simulink model "CusakisME4901arcs2"  (R2013a)
settings: Solver=ode4  StartTime=0.0  StopTime=inf  FixedStep=0.01  RelTol=1e-3
InitFcn:
  | start_EEVSCube2
  | 
  | %links masses
  | 
  | m=20;%Kg
  | 
  | l=1;%meter
  | 
  | w=0.08;
  | 
  | I=(1/12)*m*(l^2); %moment of inertia
  | 
  | %estimation error
  | 
  | mn=20+m*0.05;
  | In=I+I*0.1;
  | 
  | %controls
  | 
  | a=0.7; %singularity positive gain
  | 
  | %Chaser
  | mb=100;%kg
  | lc=2;%meters
  | lb=lc/2;%meter distance 1joint to CM
  | Ib=(1/12)*mb*(lc^2+lc^2);
  | 
  | %Target
  | 
  | mt=750;%kg target mass
  | lt=1;%meter  side lenght
  | It=(1/6)*(lt^2)*mt;
  | 
  | %Target Initial Conitions
  | 
  | x_t=2;
  | y_t=2;
  | theta_t=0.7853;
  | 
  | Init_t=[x_t;y_t;theta_t;0;0;0];
  | Iinv=pinv(eye(3)*It);
StopFcn:
  | figure(1)
  | subplot(2,1,1)
  | hold on
  | plot(time,kinetic,'g')
  | grid on
  | title('Kinetic Energy vs Time')
  | xlabel('Time')
  | ylabel('Kinetic Energy')
  | hold off
  | 
  | subplot(2,1,2)
  | hold on
  | plot(time,power,'g')
  | grid on
  | title('Power Consumption vs Time')
  | xlabel('Time')
  | ylabel('Power')
  | hold off
  | 
  | chasermapping=[-1,1;-1,-1;1,-1;1,1;-1,1];
  | targetmapping=[1.293,2;2,2.707;2.707,2;2,1.293;1.293,2];
  | 
  | figure(3)
  | hold on
  | plot(EEstate(:,1),EEstate(:,2),'g')
  | plot(targetmapping(:,1),targetmapping(:,2),'r')
  | plot(chasermapping(:,1),chasermapping(:,2),'b')
  | grid on
  | title('End Effector Path')
  | xlabel('X Axis (m)')
  | ylabel('Y Axis (m)')
  | hold off
  | 
  | 
  | figure(4)
  | subplot(2,1,1)
  | hold on
  | plot(time,qqd(:,1),'g')
  | plot(time,qqd(:,2),'r')
  | plot(time,qqd(:,3),'b')
  | grid on
  | title('Theta vs Time')
  | xlabel('Time (sec)')
  | ylabel('Theta (rad)')
  | legend( 'Theta1 ' , ' Theta2 ' , ' Theta3')
  | hold off
  | 
  | subplot(2,1,2)
  | hold on
  | plot(time,qqd(:,4),'g')
  | plot(time,qqd(:,5),'r')
  | plot(time,qqd(:,6),'b')
  | grid on
  | legend( 'Omega1 ' , ' Omega2 ', ' Omega3 ' )
  | title('Omega vs Time')
  | xlabel('Time (sec)')
  | ylabel('Omega (rad/s)')
values from neighbouring files (symbols this model uses):
  D = sqrt((Xf(1)-Xi(1))^2+(Xf(2)-Xi(2))^2)    [Arcpaths.m]
undefined symbols (not defined in the file or in its folder): mesh_A, mesh_B, serial
libraries: instrumentlib x5, simulink x3, vrlib x2, dspinverses x1, aerolibanimutils x1
(part 1 of 4)
settings Model: Creator=Grompone  LastModifiedBy=Admin

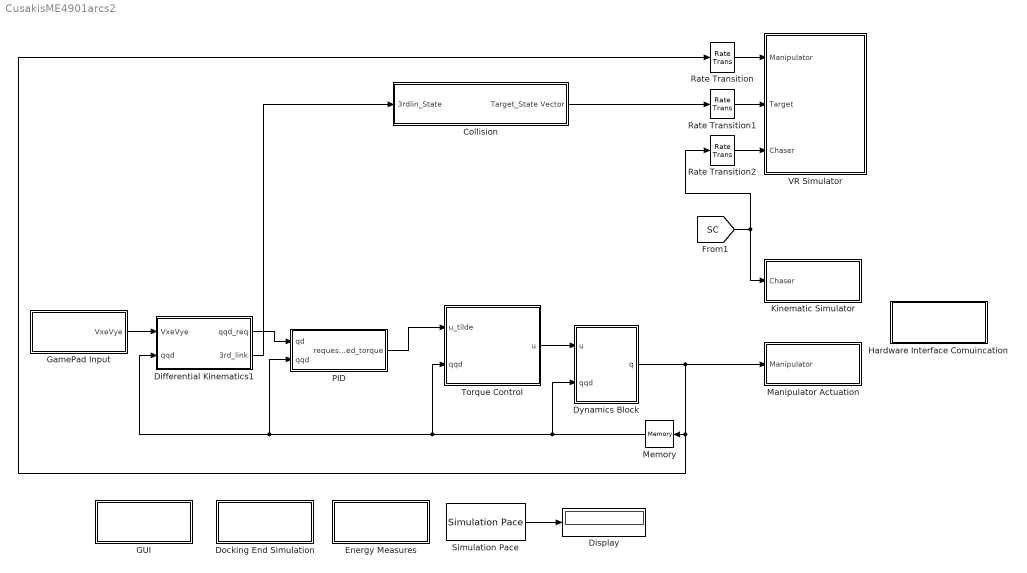
== system CusakisME4901arcs2 ==
  Collision : Subsystem
  Differential Kinematics1 : Subsystem
  Display : Display
  Docking End Simulation : Subsystem
  Dynamics Block : Subsystem
  Energy Measures : Subsystem
  GUI : Subsystem
  GamePad Input : Subsystem
  Hardware Interface Comuincation : Subsystem
  Kinematic Simulator : Subsystem
  Manipulator Actuation : Subsystem
  Memory : Memory  X0=[0 0 0 0 0 0 0 0 0]'
  PID : Subsystem
  Rate Transition : RateTransition  OutPortSampleTime=0.2
  Rate Transition1 : RateTransition  OutPortSampleTime=0.2
  Rate Transition2 : RateTransition  OutPortSampleTime=0.2
  Simulation Pace : aerolibanimutils/Simulation Pace  SimulationPace=1  SleepMode=MATLAB Thread  OutputPaceError=on  SampleTime=0.01
      settings: AttributesFormatString=%<SimulationPace> sec/sec
  Torque Control : Subsystem
  VR Simulator : Subsystem
  wires:
  Torque Control/1(u) -> Dynamics Block/1(u)
  PID/1(requested_torque) -> Torque Control/1(u_tilde)
  Dynamics Block/1(q) -> Manipulator Actuation/1(Manipulator), Rate Transition/1, Memory/1
  Differential Kinematics1/1(qqd_req) -> PID/1(qd)
  GamePad Input/1(VxeVye) -> Differential Kinematics1/1(VxeVye)
  Memory/1 -> Dynamics Block/2(qqd), Torque Control/2(qqd), PID/2(qqd), Differential Kinematics1/2(qqd)
  Collision/1(Target_State Vector) -> Rate Transition1/1
  Differential Kinematics1/2(3rd_link) -> Collision/1(3rdlin_State)
  Rate Transition/1 -> VR Simulator/1(Manipulator)
  Rate Transition1/1 -> VR Simulator/2(Target)
  Rate Transition2/1 -> VR Simulator/3(Chaser)
  Simulation Pace/1 -> Display/1
  [SC] -> Rate Transition2/1, Kinematic Simulator/1(Chaser)

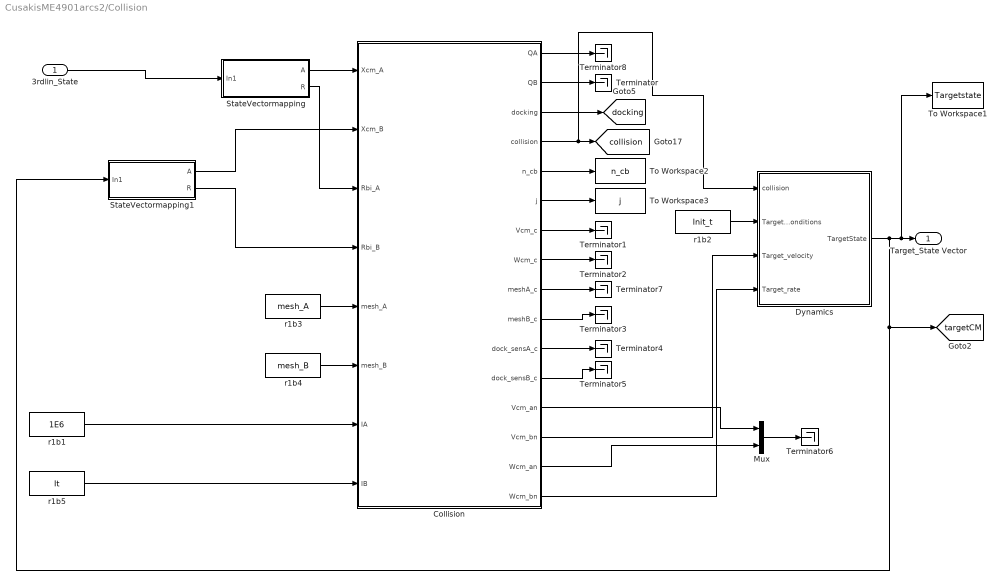
== system CusakisME4901arcs2/Collision ==
  3rdlin_State : Inport
  Collision : Subsystem  mask{mA=1e6, mB=mt, sigma=0.01, sigma_dock=0.25, dotsigma_dock=10, dock_sensA=[0.5 0 0]', dock_sensB=[0 -0.5 0]', epsilon=1}
      mask prompts: mA "Mass of body A [Kg]"; mB "Mass of body B [Kg]"; sigma "Minimum distance for contact [m]"; sigma_dock "Minimum distance for docking (must be greater than contact distance) [m]"; dotsigma_dock "Maximum relative velocity for docking [m/s]"; dock_sensA "Docking sensor position (Body RF) on body A (as [x y z]') [m]"; dock_sensB "Docking sensor position (Body RF) on body B (as [x y z]') [m]"; epsilon "Coefficent of restitution"
      mask help: This block implements collision detection and responce for two rigid bodies of general shapes.
      mask init:
      | ma_mb = [mA; 
      |          mB];
      mask Display:
      | image(imread('collision.jpeg'))
      | color('red');
      | disp('Collision \n Detection and Responce \n v.1.0.9')
      | port_label('input',1,'Xcm_A')
      | port_label('input',2,'Xcm_B')
      | port_label('input',3,'Rbi_A')
      | port_label('input',4,'Rbi_B')
      | port_label('input',5,'mesh_A')
      | port_label('input',6,'mesh_B')
      | port_label('input',7,'IA')
      | port_label('input',8,'IB')
      | 
      | port_label('output',1,'QA')
      | port_label('output',2,'QB')
      | port_label('output',3,'docking')
      | port_label('output',4,'collision')
      | port_label('output',5,'n_cb')
      | port_label('output',6,'j')
      | port_label('output',7,'Vcm_c')
      | port_label('output',8,'Wcm_c')
      | port_label('output',9,'meshA_c')
      | port_label('output',10,'meshB_c')
      | port_label('output',11,'dock_sensA_c')
      | port_label('output',12,'dock_sensB_c')
      | port_label('output',13,'Vcm_an')
      | port_label('output',14,'Vcm_bn')
      | port_label('output',15,'Wcm_an')
      | port_label('output',16,'Wcm_bn')
  Dynamics : Subsystem
  Mux : Mux  Inputs=2
  StateVectormapping : Subsystem
  StateVectormapping1 : Subsystem
  Terminator{,1..8} (9 alike) : Terminator
  To Workspace1 : ToWorkspace  VariableName=Targetstate  SampleTime=-1
  To Workspace2 : ToWorkspace  VariableName=n_cb  SampleTime=-1
  To Workspace3 : ToWorkspace  VariableName=j  SampleTime=-1
  r1b1 : Constant  Value=1E6
  r1b2 : Constant  Value=Init_t
  r1b3 : Constant  Value=mesh_A
  r1b4 : Constant  Value=mesh_B
  r1b5 : Constant  Value=It
  Target_State Vector : Outport
  tag scope: collision=global, docking=global, targetCM=global
  wires:
  Collision/3(docking) -> [docking]
  Collision/6(j) -> To Workspace3/1
  Collision/4(collision) -> Dynamics/1(collision), [collision]
  StateVectormapping/2(R) -> Collision/3(Rbi_A)
  StateVectormapping1/2(R) -> Collision/4(Rbi_B)
  r1b3/1 -> Collision/5(mesh_A)
  r1b4/1 -> Collision/6(mesh_B)
  Collision/5(n_cb) -> To Workspace2/1
  r1b1/1 -> Collision/7(IA)
  Collision/16(Wcm_bn) -> Dynamics/4(Target_rate)
  StateVectormapping1/1(A) -> Collision/2(Xcm_B)
  Collision/14(Vcm_bn) -> Dynamics/3(Target_velocity)
  r1b5/1 -> Collision/8(IB)
  StateVectormapping/1(A) -> Collision/1(Xcm_A)
  Collision/2(QB) -> Terminator/1
  Collision/7(Vcm_c) -> Terminator1/1
  Collision/8(Wcm_c) -> Terminator2/1
  Collision/9(meshA_c) -> Terminator7/1
  Collision/10(meshB_c) -> Terminator3/1
  Collision/11(dock_sensA_c) -> Terminator4/1
  Collision/12(dock_sensB_c) -> Terminator5/1
  Collision/15(Wcm_an) -> Mux/2
  Collision/13(Vcm_an) -> Mux/1
  Collision/1(QA) -> Terminator8/1
  3rdlin_State/1 -> StateVectormapping/1(In1)
  r1b2/1 -> Dynamics/2(Target_InitialConditions)
  Mux/1 -> Terminator6/1
  Dynamics/1(TargetState) -> StateVectormapping1/1(In1), [targetCM], To Workspace1/1, Target_State Vector/1

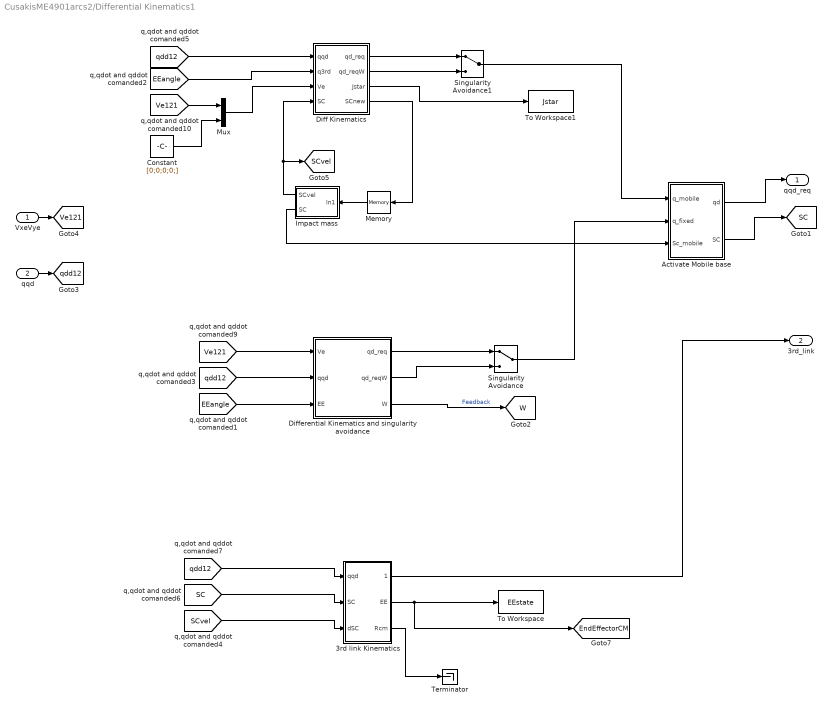
== system CusakisME4901arcs2/Differential Kinematics1 ==
  VxeVye : Inport
  qqd : Inport  Port=2
  3rd link Kinematics : MATLAB Function  TreatAsAtomicUnit=on
  Activate Mobile base : Subsystem
  Constant : Constant  Value=[0;0;0;0;]
  Diff Kinematics : MATLAB Function  TreatAsAtomicUnit=on
  Differential Kinematics and singularity avoidance : MATLAB Function  TreatAsAtomicUnit=on
  Impact mass : Subsystem
  Memory : Memory  X0=[0;0;0;0;0;0]
  Mux : Mux  Inputs=2
  Singularity Avoidance : ManualSwitch
  Singularity Avoidance1 : ManualSwitch
  Terminator : Terminator
  To Workspace : ToWorkspace  VariableName=EEstate  SampleTime=-1
  To Workspace1 : ToWorkspace  VariableName=Jstar  SampleTime=-1
  qqd_req : Outport
  3rd_link : Outport  Port=2
  tag scope: EndEffectorCM=global, SC=global, SCvel=global, Ve121=global, W=global, qdd12=global
  wires:
  Mux/1 -> Diff Kinematics/3(Ve)
  Constant/1 -> Mux/2
  Diff Kinematics/3(Jstar) -> To Workspace1/1
  Memory/1 -> Impact mass/1(In1)
  Diff Kinematics/4(SCnew) -> Memory/1
  Differential Kinematics and singularity avoidance/3(W) -> [W]  "Feedback"
  Differential Kinematics and singularity avoidance/1(qd_req) -> Singularity Avoidance/1
  Differential Kinematics and singularity avoidance/2(qd_reqW) -> Singularity Avoidance/2
  Singularity Avoidance/1 -> Activate Mobile base/2(q_fixed)
  3rd link Kinematics/1(state_3link) -> 3rd_link/1
  3rd link Kinematics/2(EE) -> [EndEffectorCM], To Workspace/1
  qqd/1 -> [qdd12]
  VxeVye/1 -> [Ve121]
  [qdd12] -> Diff Kinematics/1(qqd)
  [SC] -> 3rd link Kinematics/2(SC)
  [qdd12] -> 3rd link Kinematics/1(qqd)
  [qdd12] -> Differential Kinematics and singularity avoidance/2(qqd)
  [Ve121] -> Differential Kinematics and singularity avoidance/1(Ve)
  [EEangle] -> Diff Kinematics/2(q3rd)
  [EEangle] -> Differential Kinematics and singularity avoidance/3(EE)
  [Ve121] -> Mux/1
  Activate Mobile base/1(qd) -> qqd_req/1
  Diff Kinematics/1(qd_req) -> Singularity Avoidance1/1
  Diff Kinematics/2(qd_reqW) -> Singularity Avoidance1/2
  Singularity Avoidance1/1 -> Activate Mobile base/1(q_mobile)
  Impact mass/1(SCvel) -> [SCvel], Diff Kinematics/4(SC)
  Activate Mobile base/2(SC) -> [SC]
  Impact mass/2(SC) -> Activate Mobile base/3(Sc_mobile)
  [SCvel] -> 3rd link Kinematics/3(dSC)
  3rd link Kinematics/3(Rcm) -> Terminator/1

== system CusakisME4901arcs2/Docking End Simulation ==
  Display : Display
  Display1 : Display
  Docking and collision Detection : MATLAB Function  TreatAsAtomicUnit=on
  Memory : Memory
  Stop Simulation : Stop
  tag scope: collcount=global
  wires:
  [docking] -> Docking and collision Detection/1(Docking)
  [collision] -> Docking and collision Detection/3(Collisn)
  [D_Button] -> Docking and collision Detection/2(Dock_button)
  Docking and collision Detection/1(Stop) -> Stop Simulation/1, Display/1
  Docking and collision Detection/2(Count) -> Memory/1, [collcount], Display1/1
  Memory/1 -> Docking and collision Detection/4(Coll)

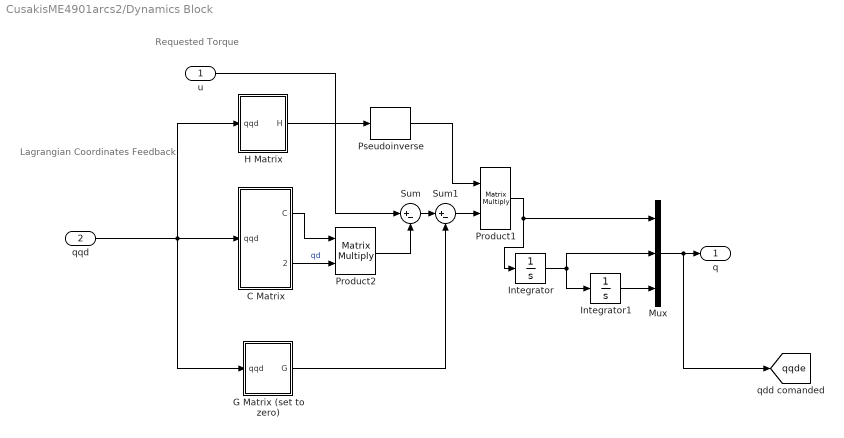
== system CusakisME4901arcs2/Dynamics Block ==
  note: Requested Torque
  note: Lagrangian Coordinates Feedback
  u : Inport
  qqd : Inport  Port=2
  C Matrix : MATLAB Function  TreatAsAtomicUnit=on
  G Matrix (set to zero) : MATLAB Function  TreatAsAtomicUnit=on
  H Matrix : MATLAB Function  TreatAsAtomicUnit=on
  Integrator : Integrator  InitialCondition=[0;0;0]
  Integrator1 : Integrator  InitialCondition=[0;0;0]
  Mux : Mux  Inputs=3
  Product1 : Product  Multiplication=Matrix(*)
  Product2 : Product  Multiplication=Matrix(*)  OutDataTypeStr=int8  LockScale=on
  Pseudoinverse : dspinverses/Pseudoinverse  wanterr=off
  Sum : Sum  Inputs=|+-
  Sum1 : Sum  Inputs=|+-
  q : Outport
  tag scope: qqde=global
  wires:
  Integrator/1 -> Mux/2, Integrator1/1
  Integrator1/1 -> Mux/3
  C Matrix/1(C) -> Product2/1
  H Matrix/1(H) -> Pseudoinverse/1
  Pseudoinverse/1 -> Product1/1
  Product1/1 -> Mux/1, Integrator/1
  Sum/1 -> Sum1/1
  Sum1/1 -> Product1/2
  G Matrix (set to zero)/1(G) -> Sum1/2
  Product2/1 -> Sum/2
  u/1 -> Sum/1
  C Matrix/2(q_dot) -> Product2/2  "qd"
  qqd/1 -> G Matrix (set to zero)/1(qqd), H Matrix/1(qqd), C Matrix/1(qqd)
  Mux/1 -> [qqde], q/1

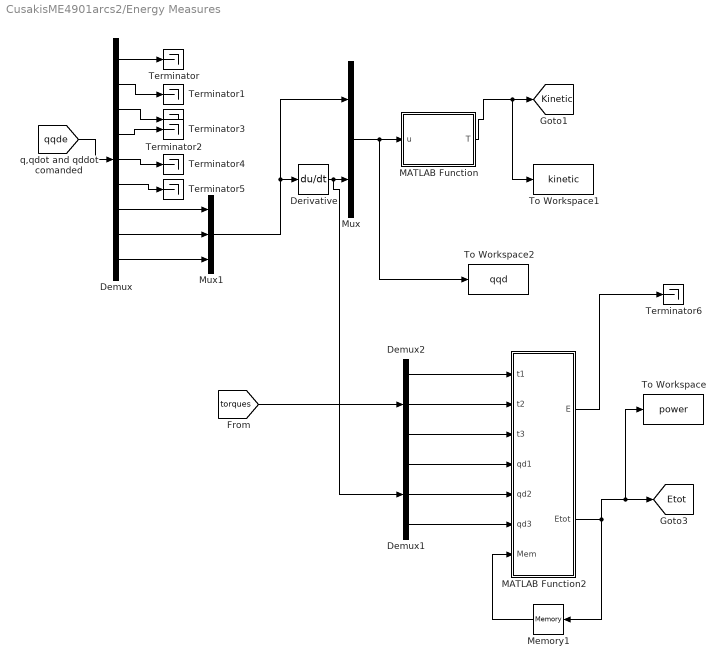
== system CusakisME4901arcs2/Energy Measures ==
  Demux : Demux  Outputs=9
  Demux1 : Demux  Outputs=3
  Demux2 : Demux  Outputs=3
  Derivative : Derivative
  MATLAB Function : MATLAB Function  TreatAsAtomicUnit=on
  MATLAB Function2 : MATLAB Function  TreatAsAtomicUnit=on
  Memory1 : Memory
  Mux : Mux  Inputs=2
  Mux1 : Mux  Inputs=3
  Terminator{,1..6} (7 alike) : Terminator
  To Workspace : ToWorkspace  VariableName=power  SampleTime=-1
  To Workspace1 : ToWorkspace  VariableName=kinetic  SampleTime=-1
  To Workspace2 : ToWorkspace  VariableName=qqd  SampleTime=-1
  tag scope: Etot=global, Kinetic=global
  wires:
  MATLAB Function/1(T) -> To Workspace1/1, [Kinetic]
  [qqde] -> Demux/1
  Demux/1 -> Terminator/1
  Demux/2 -> Terminator1/1
  Demux/3 -> Terminator2/1
  [torques] -> Demux2/1
  Memory1/1 -> MATLAB Function2/7(Mem)
  MATLAB Function2/2(Etot) -> To Workspace/1, [Etot], Memory1/1
  Demux2/1 -> MATLAB Function2/1(t1)
  Demux2/2 -> MATLAB Function2/2(t2)
  Demux2/3 -> MATLAB Function2/3(t3)
  Mux/1 -> To Workspace2/1, MATLAB Function/1(u)
  Demux/7 -> Mux1/1
  Demux/8 -> Mux1/2
  Demux/9 -> Mux1/3
  Demux/4 -> Terminator3/1
  Demux/5 -> Terminator4/1
  Demux/6 -> Terminator5/1
  Mux1/1 -> Derivative/1, Mux/1
  Derivative/1 -> Demux1/1, Mux/2
  Demux1/1 -> MATLAB Function2/4(qd1)
  Demux1/3 -> MATLAB Function2/6(qd3)
  Demux1/2 -> MATLAB Function2/5(qd2)
  MATLAB Function2/1(E) -> Terminator6/1

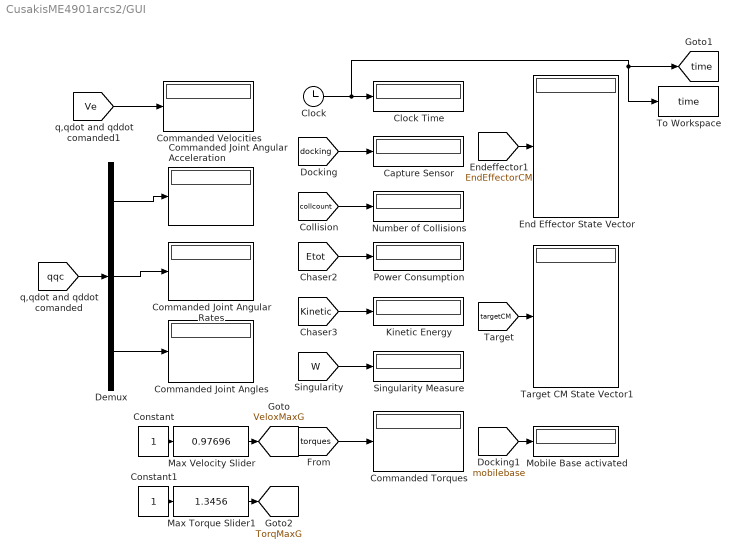
== system CusakisME4901arcs2/GUI ==
  Capture Sensor : Display
  Clock : Clock
  Clock Time : Display
  Commanded Joint Angles : Display
  Commanded Joint Angular Acceleration : Display
  Commanded Joint Angular Rates : Display
  Commanded Torques : Display
  Commanded Velocities : Display
  Constant : Constant
  Constant1 : Constant
  Demux : Demux  Outputs=3
  End Effector State Vector : Display
  Kinetic Energy : Display
  Max Torque Slider1 : simulink/Math Operations/Slider Gain  low=0  gain=1.3456  high=2
  Max Velocity Slider : simulink/Math Operations/Slider Gain  low=0  gain=0.97696  high=2
  Mobile Base activated : Display
  Number of Collisions : Display
  Power Consumption : Display
  Singularity Measure : Display
  Target CM State Vector1 : Display
  To Workspace : ToWorkspace  VariableName=time  SampleTime=-1
  tag scope: TorqMaxG=global, VeloxMaxG=global, time=global
  wires:
  [Ve] -> Commanded Velocities/1
  [W] -> Singularity Measure/1
  [docking] -> Capture Sensor/1
  [collcount] -> Number of Collisions/1
  [qqc] -> Demux/1
  Demux/1 -> Commanded Joint Angular Acceleration/1
  Demux/2 -> Commanded Joint Angular Rates/1
  Demux/3 -> Commanded Joint Angles/1
  [targetCM] -> Target CM State Vector1/1
  [EndEffectorCM] -> End Effector State Vector/1
  [Etot] -> Power Consumption/1
  [Kinetic] -> Kinetic Energy/1
  Constant/1 -> Max Velocity Slider/1
  Max Velocity Slider/1 -> [VeloxMaxG]
  [torques] -> Commanded Torques/1
  Clock/1 -> [time], To Workspace/1, Clock Time/1
  Constant1/1 -> Max Torque Slider1/1
  Max Torque Slider1/1 -> [TorqMaxG]
  [mobilebase] -> Mobile Base activated/1

== system CusakisME4901arcs2/GamePad Input ==
  Joystick Input : vrlib/Joystick Input  joyid=1  adjustports=on  forcefeed=off
  MATLAB Function : MATLAB Function  TreatAsAtomicUnit=on
  Product : Product
  Product1 : Product
  Terminator : Terminator
  VxeVye : Outport
  tag scope: D_Button=global, EEangle=global, Ve=global
  wires:
  Joystick Input/1 -> MATLAB Function/1(Axes)
  Joystick Input/2 -> MATLAB Function/2(Buttons)
  ? -> Terminator/1
  MATLAB Function/2(but) -> [D_Button]
  MATLAB Function/3(j) -> Product1/1
  Product/1 -> VxeVye/1, [Ve]
  [VeloxMaxG] -> Product/2
  MATLAB Function/1(u) -> Product/1
  [TorqMaxG] -> Product1/2
  Product1/1 -> [EEangle]

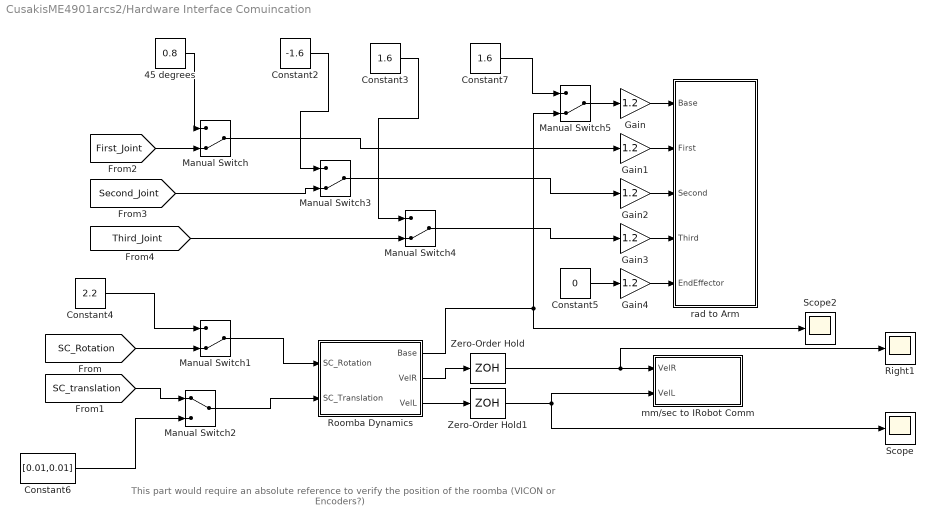
== system CusakisME4901arcs2/Hardware Interface Comuincation ==
  note: This part would require an absolute reference to verify the position of the roomba (VICON or Encoders?)
  45 degrees : Constant  Value=0.8
  Constant2 : Constant  Value=-1.6
  Constant3 : Constant  Value=1.6
  Constant4 : Constant  Value=2.2
  Constant5 : Constant  Value=0
  Constant6 : Constant  Value=[0.01,0.01]
  Constant7 : Constant  Value=1.6
  Gain{,1..4} (5 alike) : Gain  Gain=1.2
  Manual Switch{,1,3..5} (5 alike) : ManualSwitch  CurrentSetting=0
  Manual Switch2 : ManualSwitch
  Right1 : Scope
      settings: SaveName=ScopeData10
  Roomba Dynamics : Subsystem
  Scope : Scope
      settings: SaveName=ScopeData9
  Scope2 : Scope
      settings: SaveName=ScopeData11
  Zero-Order Hold : ZeroOrderHold
  Zero-Order Hold1 : ZeroOrderHold
  mm/sec to IRobot Comm : Subsystem
  rad to Arm : Subsystem
  wires:
  Constant5/1 -> Gain4/1
  [SC_Rotation] -> Manual Switch1/2
  [SC_translation] -> Manual Switch2/1
  Manual Switch2/1 -> Roomba Dynamics/2(SC_Translation)
  [Third_Joint] -> Manual Switch4/2
  Manual Switch4/1 -> Gain3/1
  [Second_Joint] -> Manual Switch3/2
  Manual Switch3/1 -> Gain2/1
  [First_Joint] -> Manual Switch/2
  Manual Switch/1 -> Gain1/1
  45 degrees/1 -> Manual Switch/1
  Constant2/1 -> Manual Switch3/1
  Constant3/1 -> Manual Switch4/1
  Constant4/1 -> Manual Switch1/1
  Constant6/1 -> Manual Switch2/2
  Constant7/1 -> Manual Switch5/1
  Roomba Dynamics/2(VelR) -> Zero-Order Hold/1
  Roomba Dynamics/3(VelL) -> Zero-Order Hold1/1
  Zero-Order Hold/1 -> Right1/1, mm/sec to IRobot Comm/1(VelR)
  Zero-Order Hold1/1 -> mm/sec to IRobot Comm/2(VelL), Scope/1
  Manual Switch5/1 -> Gain/1
  Gain/1 -> rad to Arm/1(Base)
  Gain1/1 -> rad to Arm/2(First)
  Gain2/1 -> rad to Arm/3(Second)
  Gain3/1 -> rad to Arm/4(Third)
  Gain4/1 -> rad to Arm/5(EndEffector)
  Roomba Dynamics/1(Base) -> Scope2/1, Manual Switch5/2
  Manual Switch1/1 -> Roomba Dynamics/1(SC_Rotation)

== system CusakisME4901arcs2/Kinematic Simulator ==
  Chaser : Inport
  Chaser Data : Subsystem
  Scope : Scope
      settings: SaveName=ScopeData3
  Scope2 : Scope
      settings: SaveName=ScopeData4
  chaseCM : Terminator
  tag scope: SC_Rotation=global, SC_translation=global
  wires:
  Chaser/1 -> chaseCM/1, Chaser Data/1(In1)
  Chaser Data/1(Rotation) -> [SC_Rotation], Scope/1
  Chaser Data/2(Translation) -> [SC_translation], Scope2/1

== system CusakisME4901arcs2/Manipulator Actuation ==
  Manipulator : Inport
  Manipulator Joints : Subsystem
  Scope : Scope
  Scope1 : Scope
  Scope2 : Scope
      settings: SaveName=ScopeData2
  tag scope: First_Joint=global, Second_Joint=global, Third_Joint=global
  wires:
  Manipulator/1 -> Manipulator Joints/1(In1)
  Manipulator Joints/1(Joint1) -> Scope/1, [First_Joint]
  Manipulator Joints/3(Joint4) -> [Third_Joint], Scope1/1
  Manipulator Joints/2(Joint3) -> [Second_Joint], Scope2/1

== system CusakisME4901arcs2/PID ==
  qd : Inport
  qqd : Inport  Port=2
  Add : Sum  Inputs=+++
  Demux : Demux  Outputs=3
  Derivative : Derivative
  Gain : Gain
  Gain1 : Gain
  Gain2 : Gain
  Integrator : Integrator  InitialCondition=[0; 0; 0]
  Mux : Mux  Inputs=3
  Sum : Sum  Inputs=|+-
  Sum1 : Sum  Inputs=|+-
  Terminator : Terminator
  requested_torque : Outport
  tag scope: qqc=global
  wires:
  qqd/1 -> Demux/1
  Demux/2 -> Sum/2
  Demux/1 -> Terminator/1
  Sum/1 -> Gain/1
  qd/1 -> Derivative/1, Integrator/1, Sum/1
  Gain/1 -> Mux/2, Add/2
  Sum1/1 -> Gain1/1
  Demux/3 -> Sum1/2
  Add/1 -> requested_torque/1
  Mux/1 -> [qqc]
  Gain1/1 -> Mux/3, Add/3  "Feedback"
  Integrator/1 -> Sum1/1
  Gain2/1 -> Add/1, Mux/1
  Derivative/1 -> Gain2/1

== system CusakisME4901arcs2/Torque Control ==
  u_tilde : Inport
  qqd : Inport  Port=2
  C Matrix : MATLAB Function  TreatAsAtomicUnit=on
  C*q : Product  Multiplication=Matrix(*)
  G Matrix (set zero) : MATLAB Function  TreatAsAtomicUnit=on
  H Matrix : MATLAB Function  TreatAsAtomicUnit=on
  H*u : Product  Multiplication=Matrix(*)
  Subtract : Sum  Inputs=+++
  u : Outport
  tag scope: torques=global
  wires:
  H*u/1 -> Subtract/1
  Subtract/1 -> [torques], u/1
  C*q/1 -> Subtract/2
  C Matrix/1(C) -> C*q/1
  G Matrix (set zero)/1(G) -> Subtract/3
  C Matrix/2(q_dot) -> C*q/2  "qd"
  u_tilde/1 -> H*u/2
  H Matrix/1(H) -> H*u/1
  qqd/1 -> H Matrix/1(qqd), C Matrix/1(qqd), G Matrix (set zero)/1(qqd)

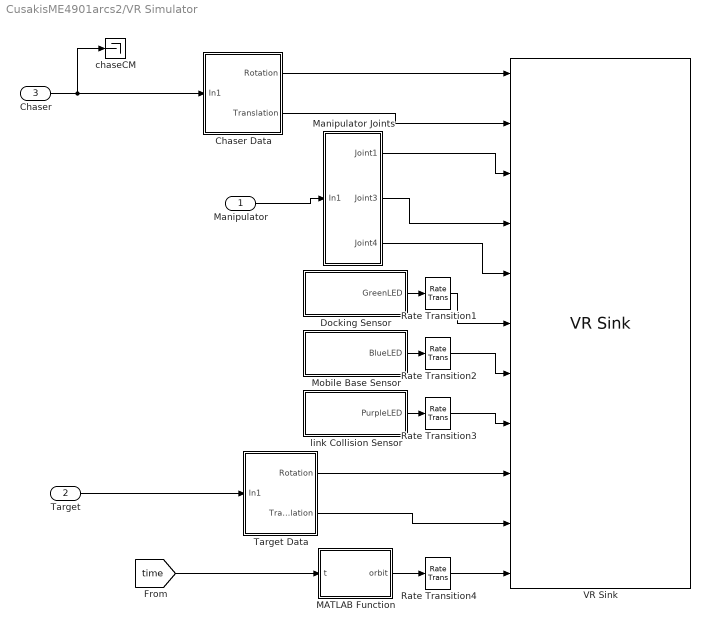
== system CusakisME4901arcs2/VR Simulator ==
  Manipulator : Inport
  Target : Inport  Port=2
  Chaser : Inport  Port=3
  Chaser Data : Subsystem
  Docking Sensor : Subsystem
  MATLAB Function : MATLAB Function  TreatAsAtomicUnit=on
  Manipulator Joints : Subsystem
  Mobile Base Sensor : Subsystem
  Rate Transition{1..4} (4 alike) : RateTransition  OutPortSampleTime=0.2
  Target Data : Subsystem
  VR Sink : vrlib/VR Sink  InstantiateOnLoad=on  SampleTime=0.2  ViewEnable=on  RemoteChange=off  RemoteView=off  FieldsWritten=CHASER.rotation.4.1.1.double#CHASER.translation.3.1.1.double#Joint1.rotation.4.1.1.double#Joint2.rotation.4.1.1.double#Joint3.rotation.4.1.1.double#we.diffuseColor.3.1.1.double#g.diffuseColor.3.1.1.double#Cl.diffuseColor.3.1.1.double#TARGET.rotation.4.1.1.double#TARGET.translation.3.1.1.double#Otherview.translation.3.1.1.double  WorldFileName=final1b.wrl  AutoView=off  VideoDimensions=[]  AllowVariableSize=off
  chaseCM : Terminator
  link Collision Sensor : Subsystem
  wires:
  Manipulator/1 -> Manipulator Joints/1(In1)
  Target/1 -> Target Data/1(In1)
  [time] -> MATLAB Function/1(t)
  Chaser/1 -> chaseCM/1, Chaser Data/1(In1)
  Chaser Data/1(Rotation) -> VR Sink/1
  Chaser Data/2(Translation) -> VR Sink/2
  Manipulator Joints/1(Joint1) -> VR Sink/3
  Manipulator Joints/3(Joint4) -> VR Sink/5
  Target Data/1(Rotation) -> VR Sink/9
  Target Data/2(Translation) -> VR Sink/10
  MATLAB Function/1(orbit) -> Rate Transition4/1
  link Collision Sensor/1(PurpleLED) -> Rate Transition3/1
  Docking Sensor/1(GreenLED) -> Rate Transition1/1
  Mobile Base Sensor/1(BlueLED) -> Rate Transition2/1
  Manipulator Joints/2(Joint3) -> VR Sink/4
  Rate Transition1/1 -> VR Sink/6
  Rate Transition2/1 -> VR Sink/7
  Rate Transition3/1 -> VR Sink/8
  Rate Transition4/1 -> VR Sink/11

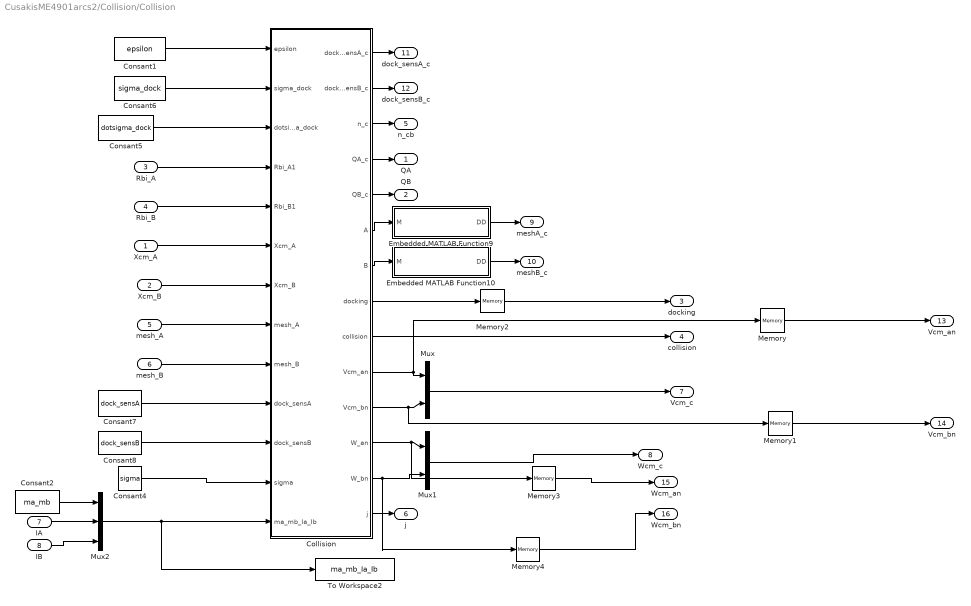
== system CusakisME4901arcs2/Collision/Collision ==
  Xcm_A : Inport
  Xcm_B : Inport  Port=2
  Rbi_A : Inport  Port=3
  Rbi_B : Inport  Port=4
  mesh_A : Inport  Port=5
  mesh_B : Inport  Port=6
  IA : Inport  Port=7
  IB : Inport  Port=8
  Collision : MATLAB Function  TreatAsAtomicUnit=on
  Consant1 : Constant  Value=epsilon
  Consant2 : Constant  Value=ma_mb
  Consant4 : Constant  Value=sigma
  Consant5 : Constant  Value=dotsigma_dock
  Consant6 : Constant  Value=sigma_dock
  Consant7 : Constant  Value=dock_sensA
  Consant8 : Constant  Value=dock_sensB
  Embedded MATLAB Function10 : MATLAB Function  TreatAsAtomicUnit=on
  Embedded MATLAB Function9 : MATLAB Function  TreatAsAtomicUnit=on
  Memory{,1,3..4} (4 alike) : Memory  X0=zeros(3,1)
  Memory2 : Memory
  Mux : Mux  Inputs=2
  Mux1 : Mux  Inputs=2
  Mux2 : Mux  Inputs=3
  To Workspace2 : ToWorkspace  VariableName=ma_mb_Ia_Ib  SampleTime=-1
  QA : Outport
  QB : Outport  Port=2
  docking : Outport  Port=3
  collision : Outport  Port=4
  n_cb : Outport  Port=5
  j : Outport  Port=6
  Vcm_c : Outport  Port=7
  Wcm_c : Outport  Port=8
  meshA_c : Outport  Port=9
  meshB_c : Outport  Port=10
  dock_sensA_c : Outport  Port=11
  dock_sensB_c : Outport  Port=12
  Vcm_an : Outport  Port=13
  Vcm_bn : Outport  Port=14
  Wcm_an : Outport  Port=15
  Wcm_bn : Outport  Port=16
  wires:
  Embedded MATLAB Function9/1(DD) -> meshA_c/1
  Embedded MATLAB Function10/1(DD) -> meshB_c/1
  Collision/6(A) -> Embedded MATLAB Function9/1(M)
  Collision/7(B) -> Embedded MATLAB Function10/1(M)
  Rbi_B/1 -> Collision/5(Rbi_B1)
  Xcm_A/1 -> Collision/6(Xcm_A)
  mesh_A/1 -> Collision/8(mesh_A)
  mesh_B/1 -> Collision/9(mesh_B)
  Collision/3(n_c) -> n_cb/1
  Collision/8(docking) -> Memory2/1
  Collision/10(Vcm_an) -> Mux/1, Memory/1
  Collision/13(W_bn) -> Mux1/2, Memory4/1
  Collision/14(j) -> j/1
  Collision/9(collision) -> collision/1
  Mux/1 -> Vcm_c/1
  Mux1/1 -> Wcm_c/1
  Collision/4(QA_c) -> QA/1
  Collision/5(QB_c) -> QB/1
  Collision/11(Vcm_bn) -> Memory1/1, Mux/2
  Collision/12(W_an) -> Memory3/1, Mux1/1
  Xcm_B/1 -> Collision/7(Xcm_B)
  Collision/2(dock_sensB_c) -> dock_sensB_c/1
  Collision/1(dock_sensA_c) -> dock_sensA_c/1
  Consant4/1 -> Collision/12(sigma)
  Consant5/1 -> Collision/3(dotsigma_dock)
  Rbi_A/1 -> Collision/4(Rbi_A1)
  Consant6/1 -> Collision/2(sigma_dock)
  Consant7/1 -> Collision/10(dock_sensA)
  Consant8/1 -> Collision/11(dock_sensB)
  Consant1/1 -> Collision/1(epsilon)
  Mux2/1 -> Collision/13(ma_mb_Ia_Ib), To Workspace2/1
  Consant2/1 -> Mux2/1
  IA/1 -> Mux2/2
  IB/1 -> Mux2/3
  Memory/1 -> Vcm_an/1
  Memory1/1 -> Vcm_bn/1
  Memory3/1 -> Wcm_an/1
  Memory4/1 -> Wcm_bn/1
  Memory2/1 -> docking/1

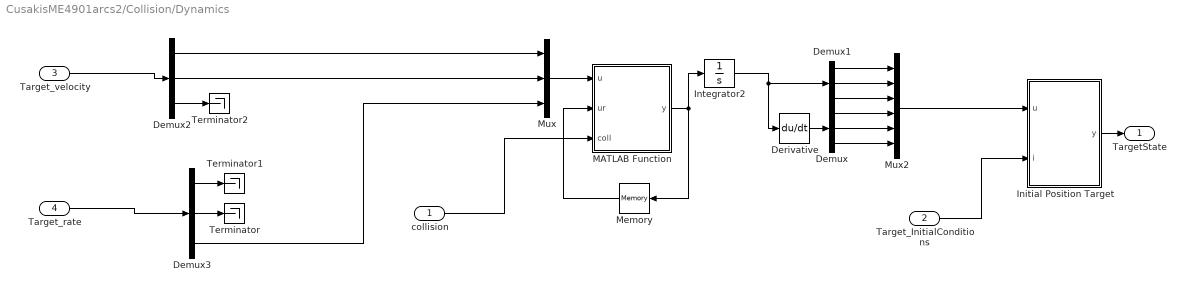
== system CusakisME4901arcs2/Collision/Dynamics ==
  collision : Inport
  Target_InitialConditions : Inport  Port=2
  Target_velocity : Inport  Port=3
  Target_rate : Inport  Port=4
  Demux{,1..3} (4 alike) : Demux  Outputs=3
  Derivative : Derivative
  Initial Position Target : MATLAB Function  TreatAsAtomicUnit=on
  Integrator2 : Integrator
  MATLAB Function : MATLAB Function  TreatAsAtomicUnit=on
  Memory : Memory  X0=[0;0;0]
  Mux : Mux  Inputs=3
  Mux2 : Mux  Inputs=6
  Terminator : Terminator
  Terminator1 : Terminator
  Terminator2 : Terminator
  TargetState : Outport
  wires:
  Target_InitialConditions/1 -> Initial Position Target/2(i)
  Initial Position Target/1(y) -> TargetState/1
  Demux2/1 -> Mux/1
  Demux2/2 -> Mux/2
  Demux3/3 -> Mux/3
  Integrator2/1 -> Derivative/1, Demux1/1
  Demux1/1 -> Mux2/1
  Demux1/2 -> Mux2/2
  Demux1/3 -> Mux2/3
  Demux/2 -> Mux2/5
  Demux/1 -> Mux2/4
  Demux/3 -> Mux2/6
  Derivative/1 -> Demux/1
  Mux2/1 -> Initial Position Target/1(u)
  Mux/1 -> MATLAB Function/1(u)
  MATLAB Function/1(y) -> Memory/1, Integrator2/1
  Memory/1 -> MATLAB Function/2(ur)
  collision/1 -> MATLAB Function/3(coll)
  Target_velocity/1 -> Demux2/1
  Target_rate/1 -> Demux3/1
  Demux3/2 -> Terminator/1
  Demux3/1 -> Terminator1/1
  Demux2/3 -> Terminator2/1

== system CusakisME4901arcs2/Collision/StateVectormapping ==
  In1 : Inport
  Rotation MAtrix1 : MATLAB Function  TreatAsAtomicUnit=on
  A : Outport
  R : Outport  Port=2
  wires:
  Rotation MAtrix1/2(R) -> R/1
  In1/1 -> Rotation MAtrix1/1(u)
  Rotation MAtrix1/1(y) -> A/1

== system CusakisME4901arcs2/Collision/StateVectormapping1 ==
  In1 : Inport
  Demux : Demux  Outputs=6
  Reshape : Reshape  OutputDimensionality=Column vector (2-D)
  Rotation MAtrix1 : MATLAB Function  TreatAsAtomicUnit=on
  A : Outport  PortDimensions=[9,1]
  R : Outport  Port=2
  wires:
  Demux/1 -> Rotation MAtrix1/1(u1)
  Demux/2 -> Rotation MAtrix1/2(u2)
  Demux/3 -> Rotation MAtrix1/3(u3)
  Demux/6 -> Rotation MAtrix1/6(u6)
  Demux/4 -> Rotation MAtrix1/4(u4)
  Demux/5 -> Rotation MAtrix1/5(u5)
  In1/1 -> Demux/1
  Rotation MAtrix1/2(R) -> R/1
  Rotation MAtrix1/1(y) -> Reshape/1
  Reshape/1 -> A/1

== system CusakisME4901arcs2/Differential Kinematics1/Activate Mobile base ==
  q_mobile : Inport
  q_fixed : Inport  Port=2
  Sc_mobile : Inport  Port=3
  MATLAB Function : MATLAB Function  TreatAsAtomicUnit=on
  Memory1 : Memory
  SC_fixed : Constant  Value=[0;0;0;0;0;0]
  Switch1 : Switch  Criteria=u2 ~= 0
  Switch2 : Switch  Criteria=u2 ~= 0
  qd : Outport
  SC : Outport  Port=2
  tag scope: mobilebase=global
  wires:
  [D_Button] -> MATLAB Function/1(but)
  Memory1/1 -> MATLAB Function/2(bo)
  MATLAB Function/1(y) -> Memory1/1, Switch1/2, Switch2/2, [mobilebase]
  q_mobile/1 -> Switch1/1
  q_fixed/1 -> Switch1/3
  Switch1/1 -> qd/1
  Sc_mobile/1 -> Switch2/1
  SC_fixed/1 -> Switch2/3
  Switch2/1 -> SC/1

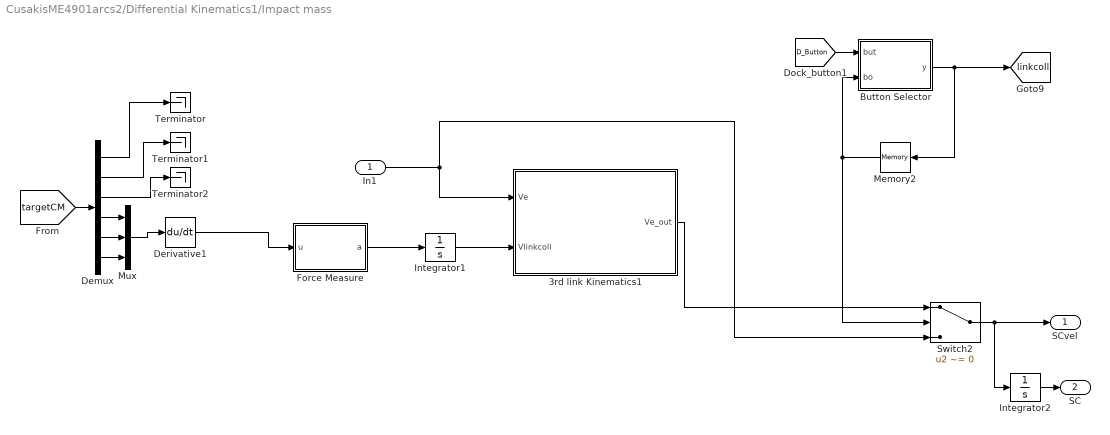
== system CusakisME4901arcs2/Differential Kinematics1/Impact mass ==
  In1 : Inport
  3rd link Kinematics1 : MATLAB Function  TreatAsAtomicUnit=on
  Button Selector : MATLAB Function  TreatAsAtomicUnit=on
  Demux : Demux  Outputs=6
  Derivative1 : Derivative  CoefficientInTFapproximation=Inf
  Force Measure : MATLAB Function  TreatAsAtomicUnit=on
  Integrator1 : Integrator  InitialCondition=[0;0;0;0;0;0]
  Integrator2 : Integrator  InitialCondition=[0;0;0;0;0;0]
  Memory2 : Memory
  Mux : Mux  Inputs=3
  Switch2 : Switch  Criteria=u2 ~= 0
  Terminator : Terminator
  Terminator1 : Terminator
  Terminator2 : Terminator
  SCvel : Outport
  SC : Outport  Port=2
  tag scope: linkcoll=global
  wires:
  Integrator1/1 -> 3rd link Kinematics1/2(Vlinkcoll)
  In1/1 -> Switch2/3, 3rd link Kinematics1/1(Ve)
  3rd link Kinematics1/1(Ve_out) -> Switch2/1
  Force Measure/1(a) -> Integrator1/1
  Derivative1/1 -> Force Measure/1(u)
  [targetCM] -> Demux/1
  Mux/1 -> Derivative1/1
  Demux/4 -> Mux/1
  Demux/5 -> Mux/2
  Demux/6 -> Mux/3
  [D_Button] -> Button Selector/1(but)
  Memory2/1 -> Switch2/2, Button Selector/2(bo)
  Button Selector/1(y) -> Memory2/1, [linkcoll]
  Switch2/1 -> Integrator2/1, SCvel/1
  Integrator2/1 -> SC/1
  Demux/1 -> Terminator/1
  Demux/2 -> Terminator1/1
  Demux/3 -> Terminator2/1

== system CusakisME4901arcs2/Hardware Interface Comuincation/Roomba Dynamics ==
  SC_Rotation : Inport
  SC_Translation : Inport  Port=2
  Add : Sum
  Demux : Demux  Outputs=2
  MATLAB Function : MATLAB Function  TreatAsAtomicUnit=on
  Memory : Memory
  Memory1 : Memory  X0=[0;0]
  Memory2 : Memory
  Memory3 : Memory  X0=[0;0]
  Memory4 : Memory
  Terminator : Terminator
  Base : Outport
  VelR : Outport  Port=2
  VelL : Outport  Port=3
  wires:
  SC_Translation/1 -> MATLAB Function/1(SCtranslation)
  Memory/1 -> MATLAB Function/4(timer)
  MATLAB Function/2(timem) -> Memory/1
  Memory1/1 -> MATLAB Function/5(NewPos)
  Demux/1 -> VelR/1
  Demux/2 -> VelL/1
  SC_Rotation/1 -> Add/2
  Add/1 -> Base/1
  MATLAB Function/3(NP) -> Memory1/1
  Memory2/1 -> MATLAB Function/6(basem)
  Memory3/1 -> MATLAB Function/3(Velm)
  MATLAB Function/1(Vel) -> Memory3/1, Demux/1
  MATLAB Function/4(base) -> Memory2/1
  MATLAB Function/6(enable) -> Terminator/1
  MATLAB Function/5(baseout) -> Memory4/1, Add/1
  Memory4/1 -> MATLAB Function/2(baseoutm)

== system CusakisME4901arcs2/Hardware Interface Comuincation/mm//sec to IRobot Comm ==
  VelR : Inport
  VelL : Inport  Port=2
  Constant : Constant  Value=128  OutDataTypeStr=uint8
  Constant1 : Constant  Value=131  OutDataTypeStr=uint8
  Constant2 : Constant  Value=145  OutDataTypeStr=uint8
  MATLAB Function : MATLAB Function  TreatAsAtomicUnit=on
  Mux : Mux  Inputs=7
  Rate Transition : RateTransition  OutPortSampleTime=1
  Subsystem : Subsystem
  wires:
  MATLAB Function/1(HiR) -> Mux/4
  MATLAB Function/2(LoR) -> Mux/5
  MATLAB Function/3(HiL) -> Mux/6
  MATLAB Function/4(LoL) -> Mux/7
  VelR/1 -> MATLAB Function/1(VelR)
  VelL/1 -> MATLAB Function/2(VelL)
  Constant/1 -> Mux/1
  Constant1/1 -> Mux/2
  Constant2/1 -> Mux/3
  Mux/1 -> Rate Transition/1
  Rate Transition/1 -> Subsystem/1(In1)

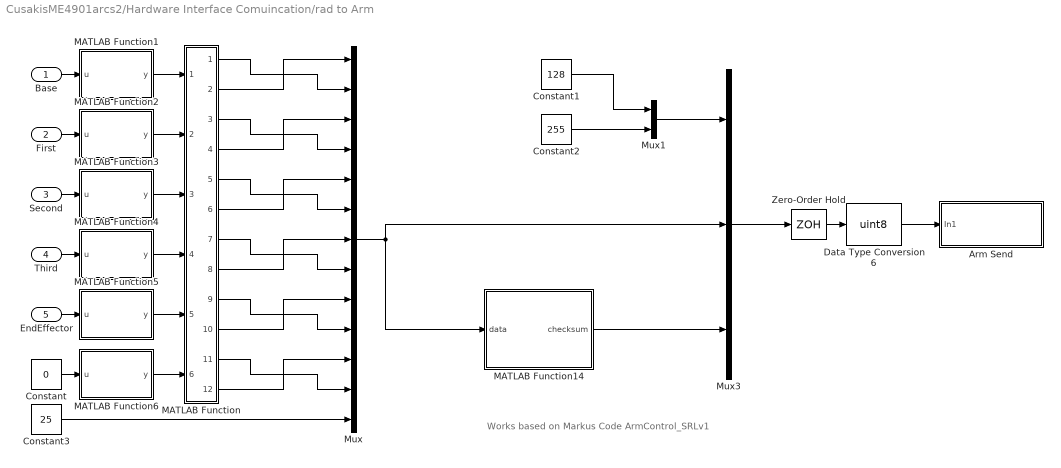
== system CusakisME4901arcs2/Hardware Interface Comuincation/rad to Arm ==
  note: Works based on Markus Code ArmControl_SRLv1
  Base : Inport
  First : Inport  Port=2
  Second : Inport  Port=3
  Third : Inport  Port=4
  EndEffector : Inport  Port=5
  Arm Send : Subsystem
  Constant : Constant  Value=0  OutDataTypeStr=uint8
  Constant1 : Constant  Value=128  OutDataTypeStr=uint8
  Constant2 : Constant  Value=255  OutDataTypeStr=uint8
  Constant3 : Constant  Value=25  OutDataTypeStr=uint8
  Data Type Conversion6 : DataTypeConversion  OutDataTypeStr=uint8
  MATLAB Function : MATLAB Function  TreatAsAtomicUnit=on
  MATLAB Function1 : MATLAB Function  TreatAsAtomicUnit=on
  MATLAB Function14 : MATLAB Function  TreatAsAtomicUnit=on
  MATLAB Function2 : MATLAB Function  TreatAsAtomicUnit=on
  MATLAB Function3 : MATLAB Function  TreatAsAtomicUnit=on
  MATLAB Function4 : MATLAB Function  TreatAsAtomicUnit=on
  MATLAB Function5 : MATLAB Function  TreatAsAtomicUnit=on
  MATLAB Function6 : MATLAB Function  TreatAsAtomicUnit=on
  Mux : Mux  Inputs=13
  Mux1 : Mux  Inputs=2
  Mux3 : Mux  Inputs=3
  Zero-Order Hold : ZeroOrderHold  SampleTime=0.01
  wires:
  EndEffector/1 -> MATLAB Function5/1(u)
  First/1 -> MATLAB Function2/1(u)
  Second/1 -> MATLAB Function3/1(u)
  Third/1 -> MATLAB Function4/1(u)
  Base/1 -> MATLAB Function1/1(u)
  Constant/1 -> MATLAB Function6/1(u)
  Constant1/1 -> Mux1/1
  Constant2/1 -> Mux1/2
  Constant3/1 -> Mux/13
  MATLAB Function14/1(checksum) -> Mux3/3
  Mux/1 -> Mux3/2, MATLAB Function14/1(data)
  Mux1/1 -> Mux3/1
  Data Type Conversion6/1 -> Arm Send/1(In1)
  MATLAB Function/2(LoBase) -> Mux/1
  MATLAB Function/4(LoM1) -> Mux/3
  MATLAB Function/6(LoM2) -> Mux/5
  MATLAB Function/8(LoM3) -> Mux/7
  MATLAB Function/10(LoEnd) -> Mux/9
  MATLAB Function/12(LoO) -> Mux/11
  MATLAB Function/1(HiBase) -> Mux/2
  MATLAB Function/3(HiM1) -> Mux/4
  MATLAB Function/5(HiM2) -> Mux/6
  MATLAB Function/7(HiM3) -> Mux/8
  MATLAB Function/9(HiEnd) -> Mux/10
  MATLAB Function/11(HiO) -> Mux/12
  MATLAB Function1/1(y) -> MATLAB Function/1(Base)
  MATLAB Function2/1(y) -> MATLAB Function/2(M1)
  MATLAB Function3/1(y) -> MATLAB Function/3(M2)
  MATLAB Function4/1(y) -> MATLAB Function/4(M3)
  MATLAB Function5/1(y) -> MATLAB Function/5(End)
  MATLAB Function6/1(y) -> MATLAB Function/6(other)
  Mux3/1 -> Zero-Order Hold/1
  Zero-Order Hold/1 -> Data Type Conversion6/1

== system CusakisME4901arcs2/Kinematic Simulator/Chaser Data ==
  In1 : Inport
  Demux2 : Demux  Outputs=6
  Gain : Gain  Gain=-1
  Mux : Mux  Inputs=2
  Scope{1..4} (4 alike) : Scope
      Scope1 settings: SaveName=ScopeData6
      Scope2 settings: SaveName=ScopeData5
      Scope3 settings: SaveName=ScopeData7
      Scope4 settings: SaveName=ScopeData8
  Terminator6 : Terminator
  Terminator7 : Terminator
  Terminator8 : Terminator
  Rotation : Outport
  Translation : Outport  Port=2
  wires:
  In1/1 -> Demux2/1
  Demux2/5 -> Scope2/1, Terminator7/1
  Demux2/4 -> Terminator6/1, Scope1/1
  Demux2/2 -> Gain/1
  Demux2/3 -> Scope3/1, Terminator8/1
  Mux/1 -> Translation/1
  Demux2/6 -> Rotation/1
  Demux2/1 -> Scope4/1, Mux/1
  Gain/1 -> Mux/2

== system CusakisME4901arcs2/Manipulator Actuation/Manipulator Joints ==
  In1 : Inport
  Demux1 : Demux  Outputs=9
  Terminator{,1..5} (6 alike) : Terminator
  Joint1 : Outport
  Joint3 : Outport  Port=2
  Joint4 : Outport  Port=3
  wires:
  Demux1/9 -> Joint4/1
  Demux1/8 -> Joint3/1
  Demux1/7 -> Joint1/1
  Demux1/6 -> Terminator5/1
  Demux1/5 -> Terminator4/1
  Demux1/4 -> Terminator3/1
  Demux1/3 -> Terminator2/1
  Demux1/2 -> Terminator1/1
  Demux1/1 -> Terminator/1
  In1/1 -> Demux1/1

== system CusakisME4901arcs2/VR Simulator/Chaser Data ==
  In1 : Inport
  Demux2 : Demux  Outputs=6
  Fixed rotation2 : Constant  Value=0
  Fixed rotation3 : Constant
  Gain : Gain  Gain=-1
  Gain1 : Gain  Gain=0.1
  Mux4 : Mux
  Mux5 : Mux  Inputs=3
  Terminator6 : Terminator
  Terminator7 : Terminator
  Terminator8 : Terminator
  Rotation : Outport
  Translation : Outport  Port=2
  wires:
  In1/1 -> Demux2/1
  Mux5/1 -> Gain1/1
  Demux2/5 -> Terminator7/1
  Demux2/4 -> Terminator6/1
  Demux2/2 -> Gain/1
  Fixed rotation2/1 -> Mux4/1, Mux4/3, Mux5/2
  Fixed rotation3/1 -> Mux4/2
  Demux2/3 -> Terminator8/1
  Gain1/1 -> Translation/1
  Mux4/1 -> Rotation/1
  Demux2/6 -> Mux4/4
  Demux2/1 -> Mux5/1
  Gain/1 -> Mux5/3

== system CusakisME4901arcs2/VR Simulator/Docking Sensor ==
  Fixed translation3 : Constant  Value=[0 0 0]
  Green : Constant  Value=[0.2 1 0.2]
  Rate Transition : RateTransition
  Red : Constant  Value=[1 0 0]
  Repeating Sequence Stair : simulink/Sources/Repeating Sequence Stair  OutValues=[0 1].'  tsamp=0.5  OutMin=[]  OutMax=[]  OutDataTypeStr=double  OutputDataTypeScalingMode=double  OutDataType=fixdt(0,8)  ConRadixGroup=Best Precision: Vector-wise  OutScaling=2^-12
  Switch : Switch  Criteria=u2 ~= 0
  Switch1 : Switch  Criteria=u2 ~= 0
  GreenLED : Outport
  wires:
  [docking] -> Switch/2
  Fixed translation3/1 -> Switch1/3
  Repeating Sequence Stair/1 -> Rate Transition/1
  Green/1 -> Switch/1
  Red/1 -> Switch1/1
  Switch1/1 -> Switch/3
  Rate Transition/1 -> Switch1/2
  Switch/1 -> GreenLED/1

== system CusakisME4901arcs2/VR Simulator/Manipulator Joints ==
  In1 : Inport
  Demux1 : Demux  Outputs=9
  Mux1 : Mux  Inputs=2
  Mux2 : Mux  Inputs=2
  Mux3 : Mux  Inputs=2
  Planar Joints : Constant  Value=[0;1;0]
  Terminator{,1..5} (6 alike) : Terminator
  Joint1 : Outport
  Joint3 : Outport  Port=2
  Joint4 : Outport  Port=3
  wires:
  In1/1 -> Demux1/1
  Demux1/8 -> Mux2/2
  Demux1/9 -> Mux3/2
  Demux1/7 -> Mux1/2
  Demux1/1 -> Terminator/1
  Demux1/2 -> Terminator1/1
  Demux1/3 -> Terminator2/1
  Demux1/4 -> Terminator3/1
  Demux1/5 -> Terminator4/1
  Demux1/6 -> Terminator5/1
  Planar Joints/1 -> Mux3/1, Mux2/1, Mux1/1
  Mux1/1 -> Joint1/1
  Mux2/1 -> Joint3/1
  Mux3/1 -> Joint4/1

== system CusakisME4901arcs2/VR Simulator/Mobile Base Sensor ==
  Green : Constant  Value=[0 0 0]
  Green1 : Constant  Value=[0 0 1]
  Switch : Switch  Criteria=u2 ~= 0
  BlueLED : Outport
  wires:
  Switch/1 -> BlueLED/1
  Green/1 -> Switch/1
  [mobilebase] -> Switch/2
  Green1/1 -> Switch/3

== system CusakisME4901arcs2/VR Simulator/Target Data ==
  In1 : Inport
  Demux2 : Demux  Outputs=6
  Fixed rotation2 : Constant  Value=0
  Fixed rotation3 : Constant
  Gain : Gain  Gain=-1
  Gain1 : Gain  Gain=0.1
  Mux4 : Mux
  Mux5 : Mux  Inputs=3
  Terminator6 : Terminator
  Terminator7 : Terminator
  Terminator8 : Terminator
  Rotation : Outport
  Translation : Outport  Port=2
  wires:
  Fixed rotation3/1 -> Mux4/2
  Fixed rotation2/1 -> Mux5/2, Mux4/3, Mux4/1
  Demux2/1 -> Mux5/1
  Demux2/2 -> Gain/1
  Demux2/3 -> Mux4/4
  Demux2/4 -> Terminator6/1
  Demux2/5 -> Terminator7/1
  Demux2/6 -> Terminator8/1
  Gain/1 -> Mux5/3
  Mux5/1 -> Gain1/1
  Gain1/1 -> Translation/1
  Mux4/1 -> Rotation/1
  In1/1 -> Demux2/1

== system CusakisME4901arcs2/VR Simulator/link Collision Sensor ==
  Black : Constant  Value=[0 0 0]
  Purple : Constant  Value=[1 0 1]
  Switch : Switch  Criteria=u2 ~= 0
  PurpleLED : Outport
  wires:
  Black/1 -> Switch/3
  [linkcoll] -> Switch/2
  Purple/1 -> Switch/1
  Switch/1 -> PurpleLED/1

== system CusakisME4901arcs2/Hardware Interface Comuincation/mm//sec to IRobot Comm/Subsystem ==
  In1 : Inport
  Serial Configuration : instrumentlib/Serial Configuration  Priority=-200000  ComPortMenu=<Please select a port...>  ComPort=COM4  ObjConstructor=serial('COM4');  BaudRate=57600  DataBits=8  Parity=none  StopBits=1  FlowControl=none  Timeout=10  ByteOrder=LittleEndian
  Serial Send : instrumentlib/Serial Send  ComPortMenu=<Please select a port...>  ComPort=COM4  ObjConstructor=serial('COM4');  Terminator=<none>  EnableBlockingMode=off
  wires:
  In1/1 -> Serial Send/1

== system CusakisME4901arcs2/Hardware Interface Comuincation/rad to Arm/Arm Send ==
  In1 : Inport
  Display2 : Display
  Display3 : Display
  Rate Transition : RateTransition  OutPortSampleTime=0.1
  Serial Configuration : instrumentlib/Serial Configuration  Priority=-200000  ComPortMenu=<Please select a port...>  ComPort=COM5  ObjConstructor=serial('COM5');  BaudRate=57600  DataBits=8  Parity=none  StopBits=1  FlowControl=none  Timeout=10  ByteOrder=LittleEndian
  Serial Receive : instrumentlib/Serial Receive  ComPortMenu=<Please select a port...>  ComPort=COM5  ObjConstructor=serial('COM5');  Terminator=<none>  DataSize="[1  16]"  DataType=uint8  EnableBlockingMode=off  ActionDataUnavailable=Output last received value  CustomValue=0  SampleTime=0.1
  Serial Send : instrumentlib/Serial Send  ComPortMenu=<Please select a port...>  ComPort=COM5  ObjConstructor=serial('COM5');  Terminator=<none>  EnableBlockingMode=off
  wires:
  In1/1 -> Rate Transition/1
  Rate Transition/1 -> Serial Send/1
  Serial Receive/1 -> Display2/1
  Serial Receive/2 -> Display3/1
